simulink model "getenergyleach"  (R2018a)
settings: Solver=VariableStepAuto  StartTime=0.0  StopTime=10.0  RelTol=1e-3
libraries: dspmathops x1
settings Model: Creator=janish  LastModifiedBy=janish

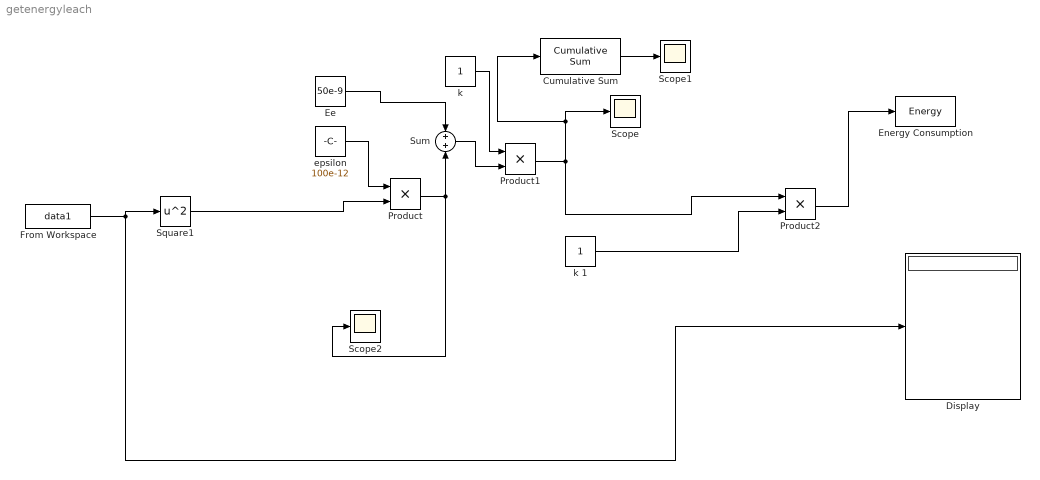
== system getenergyleach ==
  Cumulative Sum : dspmathops/Cumulative Sum  dim=Channels (running sum)  InputProcessing=Columns as channels (frame based)  reset_popup=None  roundingMode=Floor  overflowMode=off  outputDataTypeStr=Inherit: Same as accumulator  outputMin=[]  outputMax=[]  outputLastDataTypeStr=Inherit: Same as accumulator
      settings: SourceProductName=DSP System Toolbox
  Display : Display
  Ee : Constant  Value=50e-9
  "Energy Consumption " : ToWorkspace  VariableName=Energy  SampleTime=12060
      settings: MaxDataPoints=1
  From Workspace : FromWorkspace  VariableName=data1  SampleTime=12000
  Product : Product
  Product1 : Product
  Product2 : Product
  Scope : Scope
  Scope1 : Scope
  Scope2 : Scope
  Square1 : Math  Operator=square  SaturateOnIntegerOverflow=on
  Sum : Sum
  "epsilon " : Constant  Value=100e-12
  "k " : Constant
  k 1 : Constant
  wires:
  k 1/1 -> Product2/2
  From Workspace/1 -> Square1/1, Display/1
  Product2/1 -> "Energy Consumption "/1
  Square1/1 -> Product/2
  Ee/1 -> Sum/1
  Product/1 -> Scope2/1, Sum/2
  Cumulative Sum/1 -> Scope1/1
  "k "/1 -> Product1/1
  Sum/1 -> Product1/2
  "epsilon "/1 -> Product/1
  Product1/1 -> Product2/1, Scope/1, Cumulative Sum/1
